simulink model "ACC_MPC"  (R2020a)
settings: Solver=VariableStepAuto  StartTime=0.0  StopTime=20  RelTol=1e-3
libraries: mpcadaslib x1, simulink x1
settings Model: Creator=Jamie  LastModifiedBy=Jamie

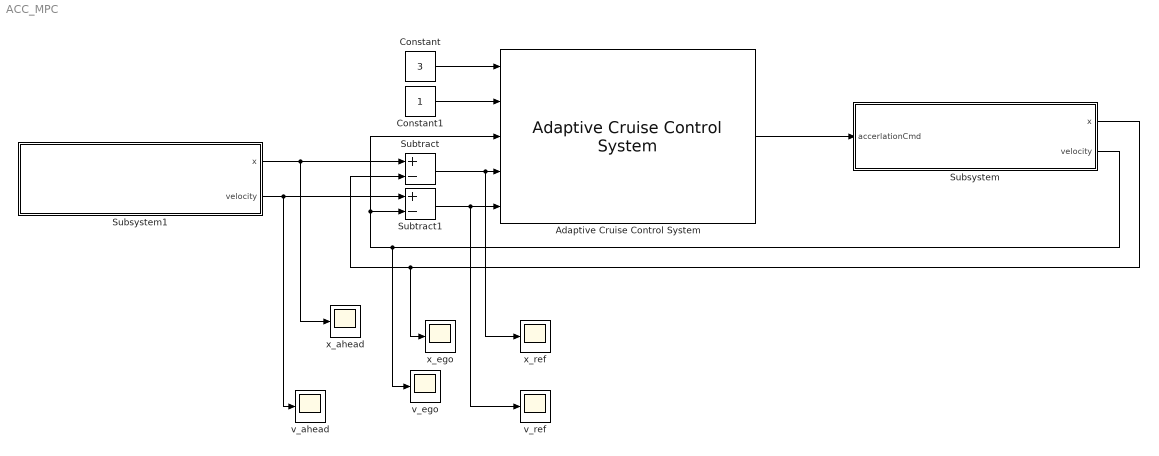
== system ACC_MPC ==
  Adaptive Cruise Control System : mpcadaslib/Adaptive Cruise Control System  EgoModel=tf(1,[0.5,1,0])  InitialEgoVelocity=0  DefaultSpacing=3  MaxVelocity=2  MinAcceleration=-3  amin_ext=off  MaxAcceleration=3  amax_ext=off  Ts=0.01  PredictionHorizon=20  ControllerBehavior=0.300  suboptimal=off  maxiter=10  datatypeopt=double  optmode=off  trackmode=off
  Constant : Constant  Value=3
  Constant1 : Constant
  Subsystem : Subsystem
  Subsystem1 : Subsystem
  Subtract : Sum  Inputs=+-
  Subtract1 : Sum  Inputs=+-
  v_ahead : Scope
  v_ego : Scope
  v_ref : Scope
  x_ahead : Scope
  x_ego : Scope
  x_ref : Scope
  wires:
  Adaptive Cruise Control System/1 -> Subsystem/1(accerlationCmd)
  Subtract/1 -> x_ref/1, Adaptive Cruise Control System/4
  Subsystem1/1(x) -> x_ahead/1, Subtract/1
  Subsystem/1(x) -> x_ego/1, Subtract/2
  Subsystem/2(velocity) -> v_ego/1, Adaptive Cruise Control System/3, Subtract1/2
  Subsystem1/2(velocity) -> v_ahead/1, Subtract1/1
  Subtract1/1 -> v_ref/1, Adaptive Cruise Control System/5
  Constant/1 -> Adaptive Cruise Control System/1
  Constant1/1 -> Adaptive Cruise Control System/2

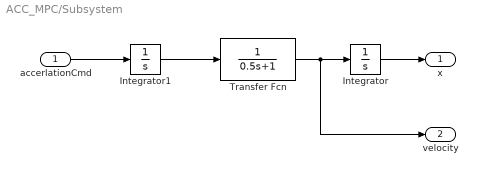
== system ACC_MPC/Subsystem ==
  accerlationCmd : Inport
  Integrator : Integrator
  Integrator1 : Integrator
  Transfer Fcn : TransferFcn  Denominator=[0.5 1]
  x : Outport
  velocity : Outport  Port=2
  wires:
  Integrator/1 -> x/1
  Transfer Fcn/1 -> velocity/1, Integrator/1
  accerlationCmd/1 -> Integrator1/1
  Integrator1/1 -> Transfer Fcn/1

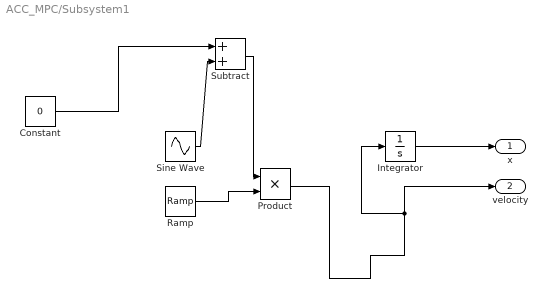
== system ACC_MPC/Subsystem1 ==
  Constant : Constant  Value=0
  Integrator : Integrator  InitialCondition=2
  Product : Product
  Ramp : simulink/Sources/Ramp  slope=0.2  start=0  InitialOutput=0
  Sine Wave : Sin  Amplitude=0.5  SampleTime=0
  Subtract : Sum
  x : Outport
  velocity : Outport  Port=2
  wires:
  Integrator/1 -> x/1
  Ramp/1 -> Product/2
  Constant/1 -> Subtract/1
  Product/1 -> velocity/1, Integrator/1
  Subtract/1 -> Product/1
  Sine Wave/1 -> Subtract/2
